simulink model "HybridCarModel"  (R2023a)
settings: Solver=VariableStepAuto  StartTime=0.0  StopTime=10.0  RelTol=1e-3
model workspace (MAT data in the model file):
  Aeff = Simulink.Parameter
  Aeff.Value = 0.0314159265359
  Aeff.DataType = 'double'
  Aeff.Complexity = 'real'
  Aeff.Dimensions = [1 1]
  Af = Simulink.Parameter
  Af.Value = 2.46
  Af.DataType = 'double'
  Af.Complexity = 'real'
  Af.Dimensions = [1 1]
  BattCapInit = Simulink.Parameter
  BattCapInit.Value = 3.18
  BattCapInit.DataType = 'double'
  BattCapInit.Complexity = 'real'
  BattCapInit.Dimensions = [1 1]
  BattChargeMax = Simulink.Parameter
  BattChargeMax.Value = 5.3
  BattChargeMax.DataType = 'double'
  BattChargeMax.Complexity = 'real'
  BattChargeMax.Dimensions = [1 1]
  BattTempBp = Simulink.Parameter
  BattTempBp.Value = [243.1 253.1 263.1 273.1 283.1 298.1 313.1]
  BattTempBp.DataType = 'double'
  BattTempBp.Complexity = 'real'
  BattTempBp.Dimensions = [1 7]
  Bx = Simulink.Parameter
  Bx.Value = 10
  Bx.DataType = 'double'
  Bx.Complexity = 'real'
  Bx.Dimensions = [1 1]
  CapLUTBp = Simulink.Parameter
  CapLUTBp.Value = [0 0.01 0.02 0.03 0.04 0.05 0.06 0.07 0.08 0.09 0.1 0.11 0.12 0.13 0.14 0.15 0.16 0.17 0.18 0.19 0.2 0.21 0.22 0.23 0.24 0.25 0.26 0.27 0.28 0.29 0.3 0.31 0.32 0.33 0.34 0.35 0.36 0.37 0.38 0.39 0.4 0.41 0.42 0.43 0.44 0.45 0.46 0.47 0.48 0.49 0.5 0.51 0.52 0.53 0.54 0.55 0.56 0.57 0.58 0.59 0.6 0.61 0.62 0.63 0.64 0.65 0.66 0.67 0.68 0.69 0.7 0.71 0.72 0.73 0.74 0.75 0.76 0.77 0.78 0.79 0.8 0.81 0.82 0.83 0.84 0.85 0.86 0.87 0.88 0.89 0.9 0.91 0.92 0.93 0.94 0.95 0.96 0.97 0.98 0.99 1]
  CapLUTBp.DataType = 'double'
  CapLUTBp.Complexity = 'real'
  CapLUTBp.Dimensions = [1 101]
  CapSOCBp = Simulink.Parameter
  CapSOCBp.Value = [0 0.2 0.4 0.6 0.8 1]
  CapSOCBp.DataType = 'double'
  CapSOCBp.Complexity = 'real'
  CapSOCBp.Dimensions = [1 6]
  CatLightOffTime = Simulink.Parameter
  CatLightOffTime.Value = 0
  CatLightOffTime.DataType = 'double'
  CatLightOffTime.Complexity = 'real'
  CatLightOffTime.Dimensions = [1 1]
  Cd = Simulink.Parameter
  Cd.Value = 0.25
  Cd.DataType = 'double'
  Cd.Complexity = 'real'
  Cd.Dimensions = [1 1]
  Cl = Simulink.Parameter
  Cl.Value = 0.1
  Cl.DataType = 'double'
  Cl.Complexity = 'real'
  Cl.Dimensions = [1 1]
  Cpm = Simulink.Parameter
  Cpm.Value = 0.1
  Cpm.DataType = 'double'
  Cpm.Complexity = 'real'
  Cpm.Dimensions = [1 1]
  Cps = Simulink.Parameter
  Cps.Value = 2
  Cps.DataType = 'double'
  Cps.Complexity = 'real'
  Cps.Dimensions = [1 1]
  CrankSpeed = Simulink.Parameter
  CrankSpeed.Value = 150
  CrankSpeed.DataType = 'double'
  CrankSpeed.Complexity = 'real'
  CrankSpeed.Dimensions = [1 1]
  Cx = Simulink.Parameter
  Cx.Value = 1.65
  Cx.DataType = 'double'
  Cx.Complexity = 'real'
  Cx.Dimensions = [1 1]
  Dx = Simulink.Parameter
  Dx.Value = 1
  Dx.DataType = 'double'
  Dx.Complexity = 'real'
  Dx.Dimensions = [1 1]
  Em = Simulink.Parameter
  Em.Value = [2.8 3.228 3.284 3.361 3.408 3.427 3.472 3.477 3.493 3.504 3.516 3.528 3.537 3.545 3.555 3.561 3.566 3.576 3.587 3.589 3.594 3.6 3.608 3.61 3.616 3.619 3.626 3.632 3.637 3.64 3.645 3.646 3.652 3.655 3.658 3.661 3.664 3.668 3.673 3.678 3.68 3.681 3.686 3.692 3.699 3.702 3.705 3.71 3.717 3.723 3.728 3.733 3.735 3.742 3.749 3.755 3.761 3.768 3.773 3.78 3.791 3.798 3.798 3.814 3.818 3.825 3.841 3.846 3.855 3.863 3.877 3.885 3.894 3.907 3.919 3.926 3.935 3.944 3.954 3.964 3.974 3.988 3.998 4.014 4.029 4.034 4.047 4.065 4.074 4.086 4.097 4.131 4.126 4.138 4.15 4.18 4.174 4.187 4.207 4.231 4.221]
  Em.DataType = 'double'
  Em.Complexity = 'real'
  Em.Dimensions = [1 101]
  EngRevLim = Simulink.Parameter
  EngRevLim.Value = 7000
  EngRevLim.DataType = 'double'
  EngRevLim.Complexity = 'real'
  EngRevLim.Dimensions = [1 1]
  EngStopStartEnable = Simulink.Parameter
  EngStopStartEnable.Value = 1
  EngStopStartEnable.DataType = 'boolean'
  EngStopStartEnable.Complexity = 'real'
  EngStopStartEnable.Dimensions = [1 1]
  EngStopTime = Simulink.Parameter
  EngStopTime.Value = 5
  EngStopTime.DataType = 'auto'
  EngStopTime.Complexity = 'real'
  EngStopTime.Dimensions = [1 1]
  Ex = Simulink.Parameter
  Ex.Value = 0.01
  Ex.DataType = 'double'
  Ex.Complexity = 'real'
  Ex.Dimensions = [1 1]
  FZMAX = Simulink.Parameter
  FZMAX.Value = 6570
  FZMAX.DataType = 'double'
  FZMAX.Complexity = 'real'
  FZMAX.Dimensions = [1 1]
  FZMIN = Simulink.Parameter
  FZMIN.Value = 0
  FZMIN.DataType = 'double'
  FZMIN.Complexity = 'real'
  FZMIN.Dimensions = [1 1]
  Fc = Simulink.Parameter
  Fc.Value = 500
  Fc.DataType = 'double'
  Fc.Complexity = 'real'
  Fc.Dimensions = [1 1]
  FsbF = Simulink.Parameter
  FsbF.Value = [-700000 -7000 -700 0 700 7000 700000]
  FsbF.DataType = 'double'
  FsbF.Complexity = 'real'
  FsbF.Dimensions = [1 7]
  FsbR = Simulink.Parameter
  FsbR.Value = [-700000 -7000 -700 0 700 7000 700000]
  FsbR.DataType = 'double'
  FsbR.Complexity = 'real'
  FsbR.Dimensions = [1 7]
  FskF = Simulink.Parameter
  FskF.Value = [-8928.57142857 -178.571428571 0 357.142857143 535.714285714 9285.71428571]
  FskF.DataType = 'double'
  FskF.Complexity = 'real'
  FskF.Dimensions = [1 6]
  FskR = Simulink.Parameter
  FskR.Value = [-5357.14285714 -107.142857143 0 214.285714286 321.428571429 5571.42857143]
  FskR.DataType = 'double'
  FskR.Complexity = 'real'
  FskR.Dimensions = [1 6]
  G = Simulink.Parameter
  G.Value = [0 1 2 3 4 5 6]
  G.DataType = 'double'
  G.Complexity = 'real'
  G.Dimensions = [1 7]
  G_o = Simulink.Parameter
  G_o.Value = 1
  G_o.DataType = 'double'
  G_o.Complexity = 'real'
  G_o.Dimensions = [1 1]
  Iyy = Simulink.Parameter
  Iyy.Value = 3000
  Iyy.DataType = 'double'
  Iyy.Complexity = 'real'
  Iyy.Dimensions = [1 1]
  Iyy_Whl = Simulink.Parameter
  Iyy_Whl.Value = 0.8
  Iyy_Whl.DataType = 'double'
  Iyy_Whl.Complexity = 'real'
  Iyy_Whl.Dimensions = [1 1]
  J = Simulink.Parameter
  J.Value = 0.01
  J.DataType = 'double'
  J.Complexity = 'real'
  J.Dimensions = [1 1]
  J1 = Simulink.Parameter
  J1.Value = 0.01
  J1.DataType = 'double'
  J1.Complexity = 'real'
  J1.Dimensions = [1 1]
  J2 = Simulink.Parameter
  J2.Value = 0.01
  J2.DataType = 'double'
  J2.Complexity = 'real'
  J2.Dimensions = [1 1]
  Jd = Simulink.Parameter
  Jd.Value = 0.01
  Jd.DataType = 'double'
  Jd.Complexity = 'real'
  Jd.Dimensions = [1 1]
  Ji = Simulink.Parameter
  Ji.Value = 0.2
  Ji.DataType = 'double'
  Ji.Complexity = 'real'
  Ji.Dimensions = [1 1]
  Jin = Simulink.Parameter
  Jin.Value = 0.05
  Jin.DataType = 'double'
  Jin.Complexity = 'real'
  Jin.Dimensions = [1 1]
  Jin_Cltch = Simulink.Parameter
  Jin_Cltch.Value = 0.2
  Jin_Cltch.DataType = 'double'
  Jin_Cltch.Complexity = 'real'
  Jin_Cltch.Dimensions = [1 1]
  Jin_Cltch2 = Simulink.Parameter
  Jin_Cltch2.Value = 0.01
  Jin_Cltch2.DataType = 'double'
  Jin_Cltch2.Complexity = 'real'
  Jin_Cltch2.Dimensions = [1 1]
  Jout = Simulink.Parameter
  Jout.Value = [0.009 0.01 0.01 0.01 0.01 0.01 0.01]
  Jout.DataType = 'double'
  Jout.Complexity = 'real'
  Jout.Dimensions = [1 7]
  Jout_Cltch = Simulink.Parameter
  Jout_Cltch.Value = 0.01
  Jout_Cltch.DataType = 'double'
  Jout_Cltch.Complexity = 'real'
  Jout_Cltch.Dimensions = [1 1]
  Jout_Cltch2 = Simulink.Parameter
  Jout_Cltch2.Value = 0.05
  Jout_Cltch2.DataType = 'double'
  Jout_Cltch2.Complexity = 'real'
  Jout_Cltch2.Dimensions = [1 1]
  Jt = Simulink.Parameter
  Jt.Value = 0.01
  Jt.DataType = 'double'
  Jt.Complexity = 'real'
  Jt.Dimensions = [1 1]
  Jw1 = Simulink.Parameter
  Jw1.Value = 0.01
  Jw1.DataType = 'double'
  Jw1.Complexity = 'real'
  Jw1.Dimensions = [1 1]
  Jw2 = Simulink.Parameter
  Jw2.Value = 0.01
  Jw2.DataType = 'double'
  Jw2.Complexity = 'real'
  Jw2.Dimensions = [1 1]
  K_c = Simulink.Parameter
  K_c.Value = 10000
  K_c.DataType = 'double'
  K_c.Complexity = 'real'
  K_c.Dimensions = [1 1]
  Lrel = Simulink.Parameter
  Lrel.Value = 0.15
  Lrel.DataType = 'double'
  Lrel.Complexity = 'real'
  Lrel.Dimensions = [1 1]
  Mass = Simulink.Parameter
  Mass.Value = 1623
  Mass.DataType = 'double'
  Mass.Complexity = 'real'
  Mass.Dimensions = [1 1]
  N = Simulink.Parameter
  N.Value = [1 4.212 2.637 1.8 1.386 1 0.772]
  N.DataType = 'double'
  N.Complexity = 'real'
  N.Dimensions = [1 7]
  NCyl = Simulink.Parameter
  NCyl.Value = 4
  NCyl.DataType = 'double'
  NCyl.Complexity = 'real'
  NCyl.Dimensions = [1 1]
  NF = Simulink.Parameter
  NF.Value = 2
  NF.DataType = 'double'
  NF.Complexity = 'real'
  NF.Dimensions = [1 1]
  NR = Simulink.Parameter
  NR.Value = 2
  NR.DataType = 'double'
  NR.Complexity = 'real'
  NR.Dimensions = [1 1]
  N_P4 = Simulink.Parameter
  N_P4.Value = 4.1
  N_P4.DataType = 'double'
  N_P4.Complexity = 'real'
  N_P4.Dimensions = [1 1]
  N_idle = Simulink.Parameter
  N_idle.Value = 750
  N_idle.DataType = 'double'
  N_idle.Complexity = 'real'
  N_idle.Dimensions = [1 1]
  Ndiff = Simulink.Parameter
  Ndiff.Value = 3.32
  Ndiff.DataType = 'double'
  Ndiff.Complexity = 'real'
  Ndiff.Dimensions = [1 1]
  Ndiff_P4 = Simulink.Parameter
  Ndiff_P4.Value = 4.1
  Ndiff_P4.DataType = 'double'
  Ndiff_P4.Complexity = 'real'
  Ndiff_P4.Dimensions = [1 1]
  Ndisk = Simulink.Parameter
  Ndisk.Value = 1
  Ndisk.DataType = 'double'
  Ndisk.Complexity = 'real'
  Ndisk.Dimensions = [1 1]
  Ndisks = Simulink.Parameter
  Ndisks.Value = 4
  Ndisks.DataType = 'double'
  Ndisks.Complexity = 'real'
  Ndisks.Dimensions = [1 1]
  Np = Simulink.Parameter
  Np.Value = 1
  Np.DataType = 'double'
  Np.Complexity = 'real'
  Np.Dimensions = [1 1]
  Ns = Simulink.Parameter
  Ns.Value = 72
  Ns.DataType = 'double'
  Ns.Complexity = 'real'
  Ns.Dimensions = [1 1]
  Pabs = Simulink.Parameter
  Pabs.Value = 101325
  Pabs.DataType = 'double'
  Pabs.Complexity = 'real'
  Pabs.Dimensions = [1 1]
  Plimit = Simulink.Parameter
  Plimit.Value = 30000
  Plimit.DataType = 'double'
  Plimit.Complexity = 'real'
  Plimit.Dimensions = [1 1]
  Press = Simulink.Parameter
  Press.Value = 7000000
  Press.DataType = 'double'
  Press.Complexity = 'real'
  Press.Dimensions = [1 1]
  Pstd = Simulink.Parameter
  Pstd.Value = 101325
  Pstd.DataType = 'double'
  Pstd.Complexity = 'real'
  Pstd.Dimensions = [1 1]
  RInt = Simulink.Parameter
  RInt.Value = [0.008846  0.009319  0.009027  0.00847  0.01032  0.01314; 0.006389  0.006554  0.005553  0.005525  0.006043  0.007805; 0.004364  0.004101  0.00406  0.003452  0.003846  0.004517; 0.002031  0.002563  0.002532  0.00246  0.002716  0.003047; 0.001443  0.001825  0.001795  0.001778  0.001924  0.002234; 0.0005603  0.0007192  0.0006887  0.0007557  0.0007355  0.001014; 0.001028  0.001338  0.001  0.001536  0.001546  0.002789]
  RInt.DataType = 'double'
  RInt.Complexity = 'real'
  RInt.Dimensions = [7 6]
  Rair = Simulink.Parameter
  Rair.Value = 287
  Rair.DataType = 'double'
  Rair.Complexity = 'real'
  Rair.Dimensions = [1 1]
  Re = Simulink.Parameter
  Re.Value = 0.327
  Re.DataType = 'double'
  Re.Complexity = 'real'
  Re.Dimensions = [1 1]
  Reff = Simulink.Parameter
  Reff.Value = 0.11
  Reff.DataType = 'double'
  Reff.Complexity = 'real'
  Reff.Dimensions = [1 1]
  Reff_LSD = Simulink.Parameter
  Reff_LSD.Value = 0.2
  Reff_LSD.DataType = 'double'
  Reff_LSD.Complexity = 'real'
  Reff_LSD.Dimensions = [1 1]
  Rm = Simulink.Parameter
  Rm.Value = 0.15
  Rm.DataType = 'double'
  Rm.Complexity = 'real'
  Rm.Dimensions = [1 1]
  Sinj = Simulink.Parameter
  Sinj.Value = 6.45161290323
  Sinj.DataType = 'double'
  Sinj.Complexity = 'real'
  Sinj.Dimensions = [1 1]
  T = Simulink.Parameter
  T.Value = 300
  T.DataType = 'double'
  T.Complexity = 'real'
  T.Dimensions = [1 1]
  T_eff_bp = Simulink.Parameter
  T_eff_bp.Value = [0 20 40 60 80 100 120 140 160 180 200]
  T_eff_bp.DataType = 'double'
  T_eff_bp.Complexity = 'real'
  T_eff_bp.Dimensions = [1 11]
  T_t = Simulink.Parameter
  T_t.Value = [200 200 200 200 190.9859317 143.2394488 114.591559 95.49296586 81.85111359 71.61972439 63.66197724 57.29577951 52.08707228 47.74648293]
  T_t.DataType = 'double'
  T_t.Complexity = 'real'
  T_t.Dimensions = [1 14]
  Tc = Simulink.Parameter
  Tc.Value = 0.02
  Tc.DataType = 'double'
  Tc.Complexity = 'real'
  Tc.Dimensions = [1 1]
  Temp_bpts = Simulink.Parameter
  Temp_bpts.Value = [313 358]
  Temp_bpts.DataType = 'double'
  Temp_bpts.Complexity = 'real'
  Temp_bpts.Dimensions = [1 2]
  Trq_bpts = Simulink.Parameter
  Trq_bpts.Value = [25 50 75 100 150 200 250]
  Trq_bpts.DataType = 'double'
  Trq_bpts.Complexity = 'real'
  Trq_bpts.Dimensions = [1 7]
  Ts = Simulink.Parameter
  Ts.Value = 0.01
  Ts.DataType = 'auto'
  Ts.Complexity = 'real'
  Ts.Dimensions = [1 1]
  Tstd = Simulink.Parameter
  Tstd.Value = 293.15
  Tstd.DataType = 'double'
  Tstd.Complexity = 'real'
  Tstd.Dimensions = [1 1]
  UNLOADED_RADIUS = Simulink.Parameter
  UNLOADED_RADIUS.Value = 0.336
  UNLOADED_RADIUS.DataType = 'double'
  UNLOADED_RADIUS.Complexity = 'real'
  UNLOADED_RADIUS.Dimensions = [1 1]
  VXLOW = Simulink.Parameter
  VXLOW.Value = 2
  VXLOW.DataType = 'double'
  VXLOW.Complexity = 'real'
  VXLOW.Dimensions = [1 1]
  Vd = Simulink.Parameter
  Vd.Value = 0.0015
  Vd.DataType = 'double'
  Vd.Complexity = 'real'
  Vd.Dimensions = [1 1]
  Vinit = Simulink.Parameter
  Vinit.Value = 650
  Vinit.DataType = 'double'
  Vinit.Complexity = 'real'
  Vinit.Dimensions = [1 1]
  aMy = Simulink.Parameter
  aMy.Value = 0.01
  aMy.DataType = 'double'
  aMy.Complexity = 'real'
  aMy.Dimensions = [1 1]
  a_CG = Simulink.Parameter
  a_CG.Value = 1.09
  a_CG.DataType = 'double'
  a_CG.Complexity = 'real'
  a_CG.Dimensions = [1 1]
  afr_stoich = Simulink.Parameter
  afr_stoich.Value = 14.6
  afr_stoich.DataType = 'double'
  afr_stoich.Complexity = 'real'
  afr_stoich.Dimensions = [1 1]
  alphaMy = Simulink.Parameter
  alphaMy.Value = 0
  alphaMy.DataType = 'double'
  alphaMy.Complexity = 'real'
  alphaMy.Dimensions = [1 1]
  b = Simulink.Parameter
  b.Value = 400
  b.DataType = 'auto'
  b.Complexity = 'real'
  b.Dimensions = [1 1]
  b1 = Simulink.Parameter
  b1.Value = 100
  b1.DataType = 'double'
  b1.Complexity = 'real'
  b1.Dimensions = [1 1]
  b1_g = Simulink.Parameter
  b1_g.Value = 0.001
  b1_g.DataType = 'double'
  b1_g.Complexity = 'real'
  b1_g.Dimensions = [1 1]
  b2 = Simulink.Parameter
  b2.Value = 100
  b2.DataType = 'double'
  b2.Complexity = 'real'
  b2.Dimensions = [1 1]
  b2_g = Simulink.Parameter
  b2_g.Value = 0.001
  b2_g.DataType = 'double'
  b2_g.Complexity = 'real'
  b2_g.Dimensions = [1 1]
  bMy = Simulink.Parameter
  bMy.Value = 0
  bMy.DataType = 'double'
  bMy.Complexity = 'real'
  bMy.Dimensions = [1 1]
  b_CG = Simulink.Parameter
  b_CG.Value = 1.7
  b_CG.DataType = 'double'
  b_CG.Complexity = 'real'
  b_CG.Dimensions = [1 1]
  b_J = Simulink.Parameter
  b_J.Value = 0.001
  b_J.DataType = 'double'
  b_J.Complexity = 'real'
  b_J.Dimensions = [1 1]
  bd = Simulink.Parameter
  bd.Value = 0.001
  bd.DataType = 'double'
  bd.Complexity = 'real'
  bd.Dimensions = [1 1]
  betaMy = Simulink.Parameter
  betaMy.Value = 1
  betaMy.DataType = 'double'
  betaMy.Complexity = 'real'
  betaMy.Dimensions = [1 1]
  bi = Simulink.Parameter
  bi.Value = 0.001
  bi.DataType = 'double'
  bi.Complexity = 'real'
  bi.Dimensions = [1 1]
  bin = Simulink.Parameter
  bin.Value = 0.003
  bin.DataType = 'double'
  bin.Complexity = 'real'
  bin.Dimensions = [1 1]
  bin_Cltch = Simulink.Parameter
  bin_Cltch.Value = 0.003
  bin_Cltch.DataType = 'double'
  bin_Cltch.Complexity = 'real'
  bin_Cltch.Dimensions = [1 1]
  bout = Simulink.Parameter
  bout.Value = [0.003 0.003 0.003 0.003 0.003 0.003 0.003]
  bout.DataType = 'double'
  bout.Complexity = 'real'
  bout.Dimensions = [1 7]
  bout_Cltch = Simulink.Parameter
  bout_Cltch.Value = 0.003
  bout_Cltch.DataType = 'double'
  bout_Cltch.Complexity = 'real'
  bout_Cltch.Dimensions = [1 1]
  br = Simulink.Parameter
  br.Value = 0.001
  br.DataType = 'double'
  br.Complexity = 'real'
  br.Dimensions = [1 1]
  bt = Simulink.Parameter
  bt.Value = 0.001
  bt.DataType = 'double'
  bt.Complexity = 'real'
  bt.Dimensions = [1 1]
  bw1 = Simulink.Parameter
  bw1.Value = 0.001
  bw1.DataType = 'double'
  bw1.Complexity = 'real'
  bw1.Dimensions = [1 1]
  bw2 = Simulink.Parameter
  bw2.Value = 0.001
  bw2.DataType = 'double'
  bw2.Complexity = 'real'
  bw2.Dimensions = [1 1]
  cMy = Simulink.Parameter
  cMy.Value = 0
  cMy.DataType = 'double'
  cMy.Complexity = 'real'
  cMy.Dimensions = [1 1]
  calEngVar.core.f_lcmd = [0 0.191691264236 0.286571334918 0.358602176328 0.434951284075 0.517809236578 0.591334464387 0.61481465749 0.61481465749 0.61481465749 0.61481465749 0.61481465749 ... (315 elements, 21x15)]
  calEngVar.core.f_tap = [0 0.526932471367 0.769562920372 0.98216383526 1.23343075188 1.55068263762 2.00046959085 2.58135491039 2.62499999998 2.62499999998 2.62499999998 2.62499999998 ... (315 elements, 21x15)]
  calEngVar.core.f_wap = [100 100 100 100 100 100 100 100 100 100 100 100 ... (315 elements, 21x15)]
  calEngVar.coreNA.f_lcmd = [0 0.191673794236 0.286480813868 0.358962317026 0.435201371684 0.516947124026 0.591296592004 0.593111529261 0.593111636908 0.593111710683 0.593111746853 0.593111755564 ... (315 elements, 21x15)]
  calEngVar.coreNA.f_tap = [0 0.527345242717 0.765291484509 0.982320090188 1.22180302541 1.45741485748 1.74956862606 2 2 2 2 2 ... (315 elements, 21x15)]
  calEngVar.coreNA.f_wap = [100 100 100 100 100 100 100 100 100 100 100 100 ... (315 elements, 21x15)]
  calEngVar.coreV.f_lcmd = [0 0.191421421753 0.286577353388 0.358588536544 0.434930146898 0.517765102071 0.591331638707 0.613375617301 0.613375617301 0.613375617301 0.613375617301 0.613375617301 ... (315 elements, 21x15)]
  calEngVar.coreV.f_tap = [0 0.527863235448 0.770830749421 0.984101116219 1.23615501042 1.5569451281 2.00979487112 2.59646979725 2.62499999998 2.62499999998 2.62499999998 2.62499999998 ... (315 elements, 21x15)]
  calEngVar.coreV.f_wap = [100 100 100 100 100 100 100 100 100 100 100 100 ... (315 elements, 21x15)]
  calEngVar.coreV2.f_lcmd = [0 0.194061751813 0.287076886738 0.359012181592 0.434856378234 0.517000734831 0.591338874186 0.631368544619 0.631368695337 0.631369347621 0.631369911122 0.631370243827 ... (315 elements, 21x15)]
  calEngVar.coreV2.f_tap = [0 0.393432535935 0.590588347082 0.770979860518 0.943173243753 1.202063296 1.55415454297 2.04859040123 2.24999782819 2.24999782819 2.24999782819 2.24999782819 ... (315 elements, 21x15)]
  calEngVar.coreV2.f_wap = [100 100 100 100 100 100 100 100 100 100 100 100 ... (315 elements, 21x15)]
  calEngVar.coreVNA.f_lcmd = [0 0.191673794234 0.286480814132 0.358962317057 0.435201376817 0.516947124415 0.5912965923 0.593111627658 0.593111729822 0.593111798315 0.593111829983 0.593111834102 ... (315 elements, 21x15)]
  calEngVar.coreVNA.f_tap = [0 0.527345232148 0.765291599327 0.982320090386 1.22180321714 1.45741495752 1.74956861419 2 2 2 2 2 ... (315 elements, 21x15)]
  calEngVar.coreVNA.f_wap = [100 100 100 100 100 100 100 100 100 100 100 100 ... (315 elements, 21x15)]
  disk_abore = Simulink.Parameter
  disk_abore.Value = 0.05
  disk_abore.DataType = 'double'
  disk_abore.Complexity = 'real'
  disk_abore.Dimensions = [1 1]
  domega_o = Simulink.Parameter
  domega_o.Value = 0
  domega_o.DataType = 'double'
  domega_o.Complexity = 'real'
  domega_o.Dimensions = [1 1]
  dw = Simulink.Parameter
  dw.Value = [0 10 20 40 60 80 100]
  dw.DataType = 'double'
  dw.Complexity = 'real'
  dw.Dimensions = [1 7]
  dzdotsF = Simulink.Parameter
  dzdotsF.Value = [-10 -1 -0.1 0 0.1 1 10]
  dzdotsF.DataType = 'double'
  dzdotsF.Complexity = 'real'
  dzdotsF.Dimensions = [1 7]
  dzdotsR = Simulink.Parameter
  dzdotsR.Value = [-10 -1 -0.1 0 0.1 1 10]
  dzdotsR.DataType = 'double'
  dzdotsR.Complexity = 'real'
  dzdotsR.Dimensions = [1 7]
  dzsF = Simulink.Parameter
  dzsF.Value = [-0.005 -0.0001 0 0.2 0.2001 0.2051]
  dzsF.DataType = 'double'
  dzsF.Complexity = 'real'
  dzsF.Dimensions = [1 6]
  dzsR = Simulink.Parameter
  dzsR.Value = [-0.005 -0.0001 0 0.2 0.2001 0.2051]
  dzsR.DataType = 'double'
  dzsR.Complexity = 'real'
  dzsR.Dimensions = [1 6]
  eff = Simulink.Parameter
  eff.Value = 98
  eff.DataType = 'double'
  eff.Complexity = 'real'
  eff.Dimensions = [1 1]
  efficiency_table = Simulink.Parameter
  efficiency_table.Value = [52  78  80  82  82  80  78  78  76  74  70; 52  78  80  82  82  80  78  78  76  74  70; 52  78  84  86  86  86  86  84  84  82  82; 52  80  86  86  88  88  88  86  86  84  84; 52  80  86  88  88  88  88  88  86  86  86; 52  80  86  88  90  90  90  90  88  88  88; 52  82  88  90  91  91  92  92  92  91  91; 52  82  88  91  91  92  93  93  93  93  93; 52  84  90  92  92  93  93  93  93  93  93; 62  86  91  93  93  93  93  93  93  93  93; 66  86  91  93  93  93  93  93  93  93  93; 70  86  92  93  93  93  93  93  93  93  93; 70  86  92  93  93  93  93  93  93  93  93; 72  86  91  93  93  93  93  93  93  93  93]
  efficiency_table.DataType = 'double'
  efficiency_table.Complexity = 'real'
  efficiency_table.Dimensions = [14 11]
  eta = Simulink.Parameter
  eta.Value = [0.95 0.95 0.95 0.95 0.95 0.95 0.95]
  eta.DataType = 'double'
  eta.Complexity = 'real'
  eta.Dimensions = [1 7]
  eta_diff = Simulink.Parameter
  eta_diff.Value = 0.98
  eta_diff.DataType = 'double'
  eta_diff.Complexity = 'real'
  eta_diff.Dimensions = [1 1]
  eta_tbl = Simulink.Parameter
  eta_tbl.Value = [0.766 0.766 0.766 0.766 0.766 0.766 0.766 0.766 0.766 0.766 0.766 0.766 ... (1078 elements, 7x11x7x2)]
  eta_tbl.DataType = 'double'
  eta_tbl.Complexity = 'real'
  eta_tbl.Dimensions = [7 11 7 2]
  f_cp_ld_bpt = Simulink.Parameter
  f_cp_ld_bpt.Value = [0 0.2 0.275 0.35 0.425 0.5 0.575 0.65 0.725 0.8 0.875 0.95 1.025 1.1 1.175 1.25]
  f_cp_ld_bpt.DataType = 'double'
  f_cp_ld_bpt.Complexity = 'real'
  f_cp_ld_bpt.Dimensions = [1 16]
  f_cp_n_bpt = Simulink.Parameter
  f_cp_n_bpt.Value = [750 1053.57142857 1357.14285714 1660.71428571 1964.28571429 2267.85714286 2571.42857143 2875 3178.57142857 3482.14285714 3785.71428571 4089.28571429 4392.85714286 4696.42857143 5000]
  f_cp_n_bpt.DataType = 'double'
  f_cp_n_bpt.Complexity = 'real'
  f_cp_n_bpt.Dimensions = [1 15]
  f_del_sa_bpt = Simulink.Parameter
  f_del_sa_bpt.Value = [0 0.75 1.5 2.25 3 3.75 4.5 5.25 6 6.75 7.5 8.25 9 9.75 10.5 11.25 12 12.75 13.5 14.25 15 15.75 16.5 17.25 18 18.75 19.5 20.25 21 21.75 22.5 23.25 24 24.75 25.5 26.25 27 27.75 28.5 29.25 30 30.75 31.5 32.25 33 33.75 34.5 35.25 36 36.75 37.5 38.25 39 39.75 40.5 41.25 42 42.75 43.5 44.25 45 45.75 46.5 47.25 48]
  f_del_sa_bpt.DataType = 'double'
  f_del_sa_bpt.Complexity = 'real'
  f_del_sa_bpt.Dimensions = [1 65]
  f_ecp = Simulink.Parameter
  f_ecp.Value = [0 0 7.19012817097 15.3709456879 19.1470470057 19.0854874367 13.5819971805 0 0 0 0 0 ... (240 elements, 16x15)]
  f_ecp.DataType = 'double'
  f_ecp.Complexity = 'real'
  f_ecp.Dimensions = [16 15]
  f_egr_areapct_cmd = Simulink.Parameter
  f_egr_areapct_cmd.Value = [0 3.448 6.897 10.34 13.79 17.24 20.69 24.14 27.59 31.03 34.48 37.93 ... (600 elements, 30x20)]
  f_egr_areapct_cmd.DataType = 'double'
  f_egr_areapct_cmd.Complexity = 'real'
  f_egr_areapct_cmd.Dimensions = [30 20]
  f_egr_areapct_nrmlzdflow_bpt = Simulink.Parameter
  f_egr_areapct_nrmlzdflow_bpt.Value = [0 0.03448 0.06897 0.1034 0.1379 0.1724 0.2069 0.2414 0.2759 0.3103 0.3448 0.3793 0.4138 0.4483 0.4828 0.5172 0.5517 0.5862 0.6207 0.6552 0.6897 0.7241 0.7586 0.7931 0.8276 0.8621 0.8966 0.931 0.9655 1]
  f_egr_areapct_nrmlzdflow_bpt.DataType = 'double'
  f_egr_areapct_nrmlzdflow_bpt.Complexity = 'real'
  f_egr_areapct_nrmlzdflow_bpt.Dimensions = [1 30]
  f_egr_areapct_pr_bpt = Simulink.Parameter
  f_egr_areapct_pr_bpt.Value = [0.5; 0.5263; 0.5526; 0.5789; 0.6053; 0.6316; 0.6579; 0.6842; 0.7105; 0.7368; 0.7632; 0.7895; 0.8158; 0.8421; 0.8684; 0.8947; 0.9211; 0.9474; 0.9737; 1]
  f_egr_areapct_pr_bpt.DataType = 'double'
  f_egr_areapct_pr_bpt.Complexity = 'real'
  f_egr_areapct_pr_bpt.Dimensions = [20 1]
  f_egr_max_stdflow = Simulink.Parameter
  f_egr_max_stdflow.Value = [74.87 74.87 74.74 74.39 73.81 72.98 71.91 70.58 68.97 67.06 64.84 62.25 59.27 55.81 51.79 47.07 36.33 24.22 12.11 0]
  f_egr_max_stdflow.DataType = 'double'
  f_egr_max_stdflow.Complexity = 'real'
  f_egr_max_stdflow.Dimensions = [1 20]
  f_egr_stdflow = Simulink.Parameter
  f_egr_stdflow.Value = [0 3.743 7.487 11.23 14.97 18.72 22.46 26.2 29.95 33.69 37.43 41.18 ... (420 elements, 21x20)]
  f_egr_stdflow.DataType = 'double'
  f_egr_stdflow.Complexity = 'real'
  f_egr_stdflow.Dimensions = [21 20]
  f_egr_stdflow_egrap_bpt = Simulink.Parameter
  f_egr_stdflow_egrap_bpt.Value = [0; 5; 10; 15; 20; 25; 30; 35; 40; 45; 50; 55; 60; 65; 70; 75; 80; 85; 90; 95; 100]
  f_egr_stdflow_egrap_bpt.DataType = 'double'
  f_egr_stdflow_egrap_bpt.Complexity = 'real'
  f_egr_stdflow_egrap_bpt.Dimensions = [21 1]
  f_egr_stdflow_pr_bpt = Simulink.Parameter
  f_egr_stdflow_pr_bpt.Value = [0.5; 0.5263; 0.5526; 0.5789; 0.6053; 0.6316; 0.6579; 0.6842; 0.7105; 0.7368; 0.7632; 0.7895; 0.8158; 0.8421; 0.8684; 0.8947; 0.9211; 0.9474; 0.9737; 1]
  f_egr_stdflow_pr_bpt.DataType = 'double'
  f_egr_stdflow_pr_bpt.Complexity = 'real'
  f_egr_stdflow_pr_bpt.Dimensions = [20 1]
  f_egrpct_cmd = Simulink.Parameter
  f_egrpct_cmd.Value = [0  0  0  0  0  0  0  0  0  0  0  0  0  0  0; 0  0  0  0  0  0  0  0  0  0  0  0  0  0  0; 0  0  0  0  0  0  0  0  0  0  0  0  0  0  0; 0  0  0  0  0  0  0  0  0  0  0  0  0  0  0; 0  0  0  0  0  0  0  0  0  0  0  0  0  0  0; 0  0  0  0  0  0  0  0  0  0  0  0  0  0  0; 0  0  0  0  0  0  0  0  0  0  0  0  0  0  0; 0  0  0  0  0  0  0  0  0  0  0  0  0  0  0; 0  0  0  0  0  0  0  0  0  0  0  0  0  0  0; 0  0  0  0  0  0  0  0  0  0  0  0  0  0  0; 0  0  0  0  0  0  0  0  0  0  0  0  0  0  0; 0  0  0  0  0  0  0  0  0  0  0  0  0  0  0; 0  0  0  0  0  0  0  0  0  0  0  0  0  0  0; 0  0  0  0  0  0  0  0  0  0  0  0  0  0  0; 0  0  0  0  0  0  0  0  0  0  0  0  0  0  0; 0  0  0  0  0  0  0  0  0  0  0  0  0  0  0]
  f_egrpct_cmd.DataType = 'double'
  f_egrpct_cmd.Complexity = 'real'
  f_egrpct_cmd.Dimensions = [16 15]
  f_egrpct_ld_bpt = Simulink.Parameter
  f_egrpct_ld_bpt.Value = [0 0.2 0.275 0.35 0.425 0.5 0.575 0.65 0.725 0.8 0.875 0.95 1.025 1.1 1.175 1.25]
  f_egrpct_ld_bpt.DataType = 'double'
  f_egrpct_ld_bpt.Complexity = 'real'
  f_egrpct_ld_bpt.Dimensions = [1 16]
  f_egrpct_n_bpt = Simulink.Parameter
  f_egrpct_n_bpt.Value = [750 1054 1357 1661 1964 2268 2571 2875 3179 3482 3786 4089 4393 4696 5000]
  f_egrpct_n_bpt.DataType = 'double'
  f_egrpct_n_bpt.Complexity = 'real'
  f_egrpct_n_bpt.Dimensions = [1 15]
  f_fric_temp_bpt = Simulink.Parameter
  f_fric_temp_bpt.Value = [274 276 278 280 282 284 286 288 290 292 294 296 298 300 302 304 306 308 310 312 314 316 318 320 322 324 326 328 330 332 334 336 338 340 342 344 346 348 350 352 354 356 358 360 362 364 366 368 370 372 374 376 378 380]
  f_fric_temp_bpt.DataType = 'double'
  f_fric_temp_bpt.Complexity = 'real'
  f_fric_temp_bpt.Dimensions = [1 54]
  f_fric_temp_mod = Simulink.Parameter
  f_fric_temp_mod.Value = [3.96 3.22 2.56 2.26 2.11 2 1.9 1.83 1.76 1.7 1.65 1.6 1.55 1.49 1.44 1.41 1.38 1.35 1.32 1.3 1.27 1.25 1.24 1.21 1.2 1.18 1.16 1.15 1.13 1.12 1.11 1.1 1.09 1.08 1.07 1.06 1.05 1.05 1.04 1.03 1.02 1.02 1.01 1.01 1 1 1 0.999 0.997 0.995 0.993 0.991 0.989 0.987]
  f_fric_temp_mod.DataType = 'double'
  f_fric_temp_mod.Complexity = 'real'
  f_fric_temp_mod.Dimensions = [1 54]
  f_icp = Simulink.Parameter
  f_icp.Value = [0 0 1 1.09273642197 2.29409401139 3.54274371837 0.947749647567 0 0 0 0 0 ... (240 elements, 16x15)]
  f_icp.DataType = 'double'
  f_icp.Complexity = 'real'
  f_icp.Dimensions = [16 15]
  f_intksys_stdflow_bpt = Simulink.Parameter
  f_intksys_stdflow_bpt.Value = [0 29.67 59.34 89.01 117.8 144.1 155.7 166 175.2 183.3 190.7 197 202.7 207.7 212.2 216.1 219.4 222.2 224.5 226.4]
  f_intksys_stdflow_bpt.DataType = 'double'
  f_intksys_stdflow_bpt.Complexity = 'real'
  f_intksys_stdflow_bpt.Dimensions = [1 20]
  f_intksys_stdflow_pr = Simulink.Parameter
  f_intksys_stdflow_pr.Value = [1 0.9789 0.9579 0.9368 0.9158 0.8947 0.8737 0.8526 0.8316 0.8105 0.7895 0.7684 0.7474 0.7263 0.7053 0.6842 0.6632 0.6421 0.6211 0.6]
  f_intksys_stdflow_pr.DataType = 'double'
  f_intksys_stdflow_pr.Complexity = 'real'
  f_intksys_stdflow_pr.Dimensions = [1 20]
  f_lamcmd = Simulink.Parameter
  f_lamcmd.Value = [1  1  1  1  1  1  1  1  1  1  1  1  1  1  1; 1  1  1  1  1  1  1  1  1  1  1  1  1  1  1; 1  1  1  1  1  1  1  1  1  1  1  1  1  1  1; 1  1  1  1  1  1  1  1  1  1  1  1  1  1  1; 1  1  1  1  1  1  1  1  1  1  1  1  1  1  1; 1  1  1  1  1  1  1  1  1  1  1  1  1  1  1; 1  1  1  1  1  1  1  1  1  1  1  1  1  1  1; 1  1  1  1  1  1  1  1  1  1  1  1  1  1  1; 1  1  1  1  1  1  1  1  1  1  1  1  1  1  1; 1  1  1  1  1  1  1  1  1  1  1  1  1  1  1; 1  1  1  1  1  1  1  1  1  1  1  1  1  1  0.978833376279; 1  1  1  1  1  0.994115442909  1  0.972947102204  0.980523305065  0.999379925377  1  0.999606769395  0.999730304812  0.995941175028  0.966904774685; 1  1  1  0.94651624294  1  0.952506105741  0.994491417815  0.906466250495  0.924122061249  0.974767007025  0.985748891861  0.982416523617  0.992900047913  0.942109771144  0.941787575943; 1  1  1  0.942  0.937279637266  0.910896768573  0.929830385386  0.839985398785  0.854904769548  0.889462296842  0.92380217143  0.919912974116  0.958707785886  0.945711085936  0.914402970615; 1  1  1  0.942  0.902  0.869287431405  0.865169352957  0.81  0.824  0.812  0.837314196571  0.85940898562  0.888506841156  0.882667105929  0.87548189152; 1  1  1  0.942  0.902  0.846  0.824  0.81  0.824  0.812  0.826  0.818  0.815209011399  0.813810193086  0.836]
  f_lamcmd.DataType = 'double'
  f_lamcmd.Complexity = 'real'
  f_lamcmd.Dimensions = [16 15]
  f_lamcmd_ld_bpt = Simulink.Parameter
  f_lamcmd_ld_bpt.Value = [0 0.2 0.275 0.35 0.425 0.5 0.575 0.65 0.725 0.8 0.875 0.95 1.025 1.1 1.175 1.25]
  f_lamcmd_ld_bpt.DataType = 'double'
  f_lamcmd_ld_bpt.Complexity = 'real'
  f_lamcmd_ld_bpt.Dimensions = [1 16]
  f_lamcmd_n_bpt = Simulink.Parameter
  f_lamcmd_n_bpt.Value = [750 1053.57142857 1357.14285714 1660.71428571 1964.28571429 2267.85714286 2571.42857143 2875 3178.57142857 3482.14285714 3785.71428571 4089.28571429 4392.85714286 4696.42857143 5000]
  f_lamcmd_n_bpt.DataType = 'double'
  f_lamcmd_n_bpt.Complexity = 'real'
  f_lamcmd_n_bpt.Dimensions = [1 15]
  f_lcmd = Simulink.Parameter
  f_lcmd.Value = [0 0.191691264236 0.286571334918 0.358602176328 0.434951284075 0.517809236578 0.591334464387 0.61481465749 0.61481465749 0.61481465749 0.61481465749 0.61481465749 ... (315 elements, 21x15)]
  f_lcmd.DataType = 'double'
  f_lcmd.Complexity = 'real'
  f_lcmd.Dimensions = [21 15]
  f_lcmd_n_bpt = Simulink.Parameter
  f_lcmd_n_bpt.Value = [750 1053.57142857 1357.14285714 1660.71428571 1964.28571429 2267.85714286 2571.42857143 2875 3178.57142857 3482.14285714 3785.71428571 4089.28571429 4392.85714286 4696.42857143 5000]
  f_lcmd_n_bpt.DataType = 'double'
  f_lcmd_n_bpt.Complexity = 'real'
  f_lcmd_n_bpt.Dimensions = [1 15]
  f_lcmd_tq_bpt = Simulink.Parameter
  f_lcmd_tq_bpt.Value = [0 15 26.3157894737 37.6315789474 48.9473684211 60.2631578947 71.5789473684 82.8947368421 94.2105263158 105.526315789 116.842105263 128.157894737 139.473684211 150.789473684 162.105263158 173.421052632 184.736842105 196.052631579 207.368421053 218.684210526 230]
  f_lcmd_tq_bpt.DataType = 'double'
  f_lcmd_tq_bpt.Complexity = 'real'
  f_lcmd_tq_bpt.Dimensions = [1 21]
  f_m_lam = Simulink.Parameter
  f_m_lam.Value = [0.94128 0.95565 0.97001 0.98437 0.99008 1.0004 0.97527 0.9549 0.92612 0.89735 0]
  f_m_lam.DataType = 'double'
  f_m_lam.Complexity = 'real'
  f_m_lam.Dimensions = [1 11]
  f_m_lam_bpt = Simulink.Parameter
  f_m_lam_bpt.Value = [0.65 0.7 0.75 0.8 0.85 0.9 0.95 1 1.05 1.1 2]
  f_m_lam_bpt.DataType = 'double'
  f_m_lam_bpt.Complexity = 'real'
  f_m_lam_bpt.Dimensions = [1 11]
  f_m_sa = Simulink.Parameter
  f_m_sa.Value = [1.0019 0.9988 0.9953 0.99173 0.98811 0.98441 0.98065 0.97682 0.97293 0.96897 0.96493 0.96083 0.95666 0.95242 0.94811 0.94373 0.93927 0.93475 0.93015 0.92548 0.92074 0.91592 0.91104 0.90608 0.90105 0.89594 0.89076 0.88551 0.88019 0.8748 0.86933 0.86379 0.85818 0.8525 0.84675 0.84093 0.83503 0.82907 0.82303 0.81693 0.81075 0.80451 0.79819 0.79181 0.78536 0.77884 0.77226 0.7656 0.75888 0.75209 0.74524 0.73832 0.73134 0.72429 0.71717 0.70999 0.70275 0.69682 0.68949 0.68303 0.67548 0.67037 0.66525 0.66014 0.65503]
  f_m_sa.DataType = 'double'
  f_m_sa.Complexity = 'real'
  f_m_sa.Dimensions = [1 65]
  f_mdot_air_corr = Simulink.Parameter
  f_mdot_air_corr.Value = [1.02156051768 1.00597426471 0.989411677851 1.0033499089 0.984591437857 0.988509040623 1.0326198627 1.02765527362 1.0134784519 0.998280021213 0.981755128787 0.967218261288 ... (400 elements, 20x20)]
  f_mdot_air_corr.DataType = 'double'
  f_mdot_air_corr.Complexity = 'real'
  f_mdot_air_corr.Dimensions = [20 20]
  f_mdot_air_corr_ld_bpt = Simulink.Parameter
  f_mdot_air_corr_ld_bpt.Value = [0.223381333333 0.285105122807 0.346828912281 0.408552701754 0.470276491228 0.532000280702 0.593724070175 0.655447859649 0.717171649123 0.778895438596 0.84061922807 0.902343017544 0.964066807018 1.02579059649 1.08751438596 1.14923817544 1.21096196491 1.27268575439 1.33440954386 1.39613333333]
  f_mdot_air_corr_ld_bpt.DataType = 'double'
  f_mdot_air_corr_ld_bpt.Complexity = 'real'
  f_mdot_air_corr_ld_bpt.Dimensions = [1 20]
  f_mdot_air_n_bpt = Simulink.Parameter
  f_mdot_air_n_bpt.Value = [750 973.6842 1197.3684 1421.0526 1644.7368 1868.4211 2092.1053 2315.7895 2539.4737 2763.1579 2986.8421 3210.5263 3434.2105 3657.8947 3881.5789 4105.2632 4328.9474 4552.6316 4776.3158 5000]
  f_mdot_air_n_bpt.DataType = 'double'
  f_mdot_air_n_bpt.Complexity = 'real'
  f_mdot_air_n_bpt.Dimensions = [1 20]
  f_mdot_intk = Simulink.Parameter
  f_mdot_intk.Value = [0 0 0 0 0 0 0 0 0 0 0 0 ... (400 elements, 20x20)]
  f_mdot_intk.DataType = 'double'
  f_mdot_intk.Complexity = 'real'
  f_mdot_intk.Dimensions = [20 20]
  f_mdot_intk_ecp_bpt = Simulink.Parameter
  f_mdot_intk_ecp_bpt.Value = [0 2.6316 5.2632 7.8947 10.5263 13.1579 15.7895 18.4211 21.0526 23.6842 26.3158 28.9474 31.5789 34.2105 36.8421 39.4737 42.1053 44.7368 47.3684 50]
  f_mdot_intk_ecp_bpt.DataType = 'double'
  f_mdot_intk_ecp_bpt.Complexity = 'real'
  f_mdot_intk_ecp_bpt.Dimensions = [1 20]
  f_mdot_trpd_bpt = Simulink.Parameter
  f_mdot_trpd_bpt.Value = [0 5.7895 11.5789 17.3684 23.1579 28.9474 34.7368 40.5263 46.3158 52.1053 57.8947 63.6842 69.4737 75.2632 81.0526 86.8421 92.6316 98.4211 104.2105 110]
  f_mdot_trpd_bpt.DataType = 'double'
  f_mdot_trpd_bpt.Complexity = 'real'
  f_mdot_trpd_bpt.Dimensions = [1 20]
  f_nv = Simulink.Parameter
  f_nv.Value = [0.64175366561 0.641419295169 0.640125365558 0.638690556197 0.644169906538 0.669178791311 0.731659452876 0.750078238889 0.750078238889 0.750078238889 0.750078238889 0.750078238889 ... (225 elements, 15x15)]
  f_nv.DataType = 'double'
  f_nv.Complexity = 'real'
  f_nv.Dimensions = [15 15]
  f_nv_n_bpt = Simulink.Parameter
  f_nv_n_bpt.Value = [750 1053.57142857 1357.14285714 1660.71428571 1964.28571429 2267.85714286 2571.42857143 2875 3178.57142857 3482.14285714 3785.71428571 4089.28571429 4392.85714286 4696.42857143 5000]
  f_nv_n_bpt.DataType = 'double'
  f_nv_n_bpt.Complexity = 'real'
  f_nv_n_bpt.Dimensions = [1 15]
  f_nv_prs_bpt = Simulink.Parameter
  f_nv_prs_bpt.Value = [31 40.6428571429 50.2857142857 59.9285714286 69.5714285714 79.2142857143 88.8571428571 98.5 108.142857143 117.785714286 127.428571429 137.071428571 146.714285714 156.357142857 166]
  f_nv_prs_bpt.DataType = 'double'
  f_nv_prs_bpt.Complexity = 'real'
  f_nv_prs_bpt.Dimensions = [1 15]
  f_sa = Simulink.Parameter
  f_sa.Value = [9.05 9.05 16.4373253582 15.3405265461 13.6074880273 9.83352189562 3.89388784387 0 0 0 0 0 ... (240 elements, 16x15)]
  f_sa.DataType = 'double'
  f_sa.Complexity = 'real'
  f_sa.Dimensions = [16 15]
  f_sa_ld_bpt = Simulink.Parameter
  f_sa_ld_bpt.Value = [0 0.2 0.275 0.35 0.425 0.5 0.575 0.65 0.725 0.8 0.875 0.95 1.025 1.1 1.175 1.25]
  f_sa_ld_bpt.DataType = 'double'
  f_sa_ld_bpt.Complexity = 'real'
  f_sa_ld_bpt.Dimensions = [1 16]
  f_sa_n_bpt = Simulink.Parameter
  f_sa_n_bpt.Value = [750 1053.57142857 1357.14285714 1660.71428571 1964.28571429 2267.85714286 2571.42857143 2875 3178.57142857 3482.14285714 3785.71428571 4089.28571429 4392.85714286 4696.42857143 5000]
  f_sa_n_bpt.DataType = 'double'
  f_sa_n_bpt.Complexity = 'real'
  f_sa_n_bpt.Dimensions = [1 15]
  f_sa_opt = Simulink.Parameter
  f_sa_opt.Value = [9.05 9.05 16.4373253582 15.3405265461 13.6074880273 9.83352189562 3.89388784387 2.22044604925e-16 2.22044604925e-16 2.22044604925e-16 2.22044604925e-16 2.22044604925e-16 ... (272 elements, 16x17)]
  f_sa_opt.DataType = 'double'
  f_sa_opt.Complexity = 'real'
  f_sa_opt.Dimensions = [16 17]
  f_startup_ect_bpt = Simulink.Parameter
  f_startup_ect_bpt.Value = [-40 0 20 50]
  f_startup_ect_bpt.DataType = 'double'
  f_startup_ect_bpt.Complexity = 'real'
  f_startup_ect_bpt.Dimensions = [1 4]
  f_startup_lambda_delta = Simulink.Parameter
  f_startup_lambda_delta.Value = [0.5 0.3 0.2 0]
  f_startup_lambda_delta.DataType = 'double'
  f_startup_lambda_delta.Complexity = 'real'
  f_startup_lambda_delta.Dimensions = [1 4]
  f_startup_lambda_delta_timecnst = Simulink.Parameter
  f_startup_lambda_delta_timecnst.Value = [90 40 12 0]
  f_startup_lambda_delta_timecnst.DataType = 'double'
  f_startup_lambda_delta_timecnst.Complexity = 'real'
  f_startup_lambda_delta_timecnst.Dimensions = [1 4]
  f_t_exh = Simulink.Parameter
  f_t_exh.Value = [739.936218766 750.584766028 772.770773797 791.235245621 803.106549716 885.862998064 920.498479307 920.498479307 920.498479307 920.498479307 920.498479307 920.498479307 ... (225 elements, 15x15)]
  f_t_exh.DataType = 'double'
  f_t_exh.Complexity = 'real'
  f_t_exh.Dimensions = [15 15]
  f_t_exh_l_bpt = Simulink.Parameter
  f_t_exh_l_bpt.Value = [0.2 0.275 0.35 0.425 0.5 0.575 0.65 0.725 0.8 0.875 0.95 1.025 1.1 1.175 1.25]
  f_t_exh_l_bpt.DataType = 'double'
  f_t_exh_l_bpt.Complexity = 'real'
  f_t_exh_l_bpt.Dimensions = [1 15]
  f_t_exh_n_bpt = Simulink.Parameter
  f_t_exh_n_bpt.Value = [750 1053.57142857 1357.14285714 1660.71428571 1964.28571429 2267.85714286 2571.42857143 2875 3178.57142857 3482.14285714 3785.71428571 4089.28571429 4392.85714286 4696.42857143 5000]
  f_t_exh_n_bpt.DataType = 'double'
  f_t_exh_n_bpt.Complexity = 'real'
  f_t_exh_n_bpt.Dimensions = [1 15]
  f_tap = Simulink.Parameter
  f_tap.Value = [0 0.526932471367 0.769562920372 0.98216383526 1.23343075188 1.55068263762 2.00046959085 2.58135491039 2.62499999998 2.62499999998 2.62499999998 2.62499999998 ... (315 elements, 21x15)]
  f_tap.DataType = 'double'
  f_tap.Complexity = 'real'
  f_tap.Dimensions = [21 15]
  f_tap_ld_bpt = Simulink.Parameter
  f_tap_ld_bpt.Value = [0 0.2 0.268421052632 0.336842105263 0.405263157895 0.473684210526 0.542105263158 0.610526315789 0.678947368421 0.747368421053 0.815789473684 0.884210526316 0.952631578947 1.02105263158 1.08947368421 1.15789473684 1.22631578947 1.29473684211 1.36315789474 1.43157894737 1.5]
  f_tap_ld_bpt.DataType = 'double'
  f_tap_ld_bpt.Complexity = 'real'
  f_tap_ld_bpt.Dimensions = [1 21]
  f_tap_n_bpt = Simulink.Parameter
  f_tap_n_bpt.Value = [750 1053.57142857 1357.14285714 1660.71428571 1964.28571429 2267.85714286 2571.42857143 2875 3178.57142857 3482.14285714 3785.71428571 4089.28571429 4392.85714286 4696.42857143 5000]
  f_tap_n_bpt.DataType = 'double'
  f_tap_n_bpt.Complexity = 'real'
  f_tap_n_bpt.Dimensions = [1 15]
  f_tm_corr = Simulink.Parameter
  f_tm_corr.Value = [0.839360054391 0.833393271885 0.82629554201 0.818442814437 0.811524387436 0.809164184856 0.814606352881 0.826887956871 0.842304598924 0.856886829014 0.869487025783 0.880530414174 ... (400 elements, 20x20)]
  f_tm_corr.DataType = 'double'
  f_tm_corr.Complexity = 'real'
  f_tm_corr.Dimensions = [20 20]
  f_tm_corr_n_bpt = Simulink.Parameter
  f_tm_corr_n_bpt.Value = [750 973.6842 1197.3684 1421.0526 1644.7368 1868.4211 2092.1053 2315.7895 2539.4737 2763.1579 2986.8421 3210.5263 3434.2105 3657.8947 3881.5789 4105.2632 4328.9474 4552.6316 4776.3158 5000]
  f_tm_corr_n_bpt.DataType = 'double'
  f_tm_corr_n_bpt.Complexity = 'real'
  f_tm_corr_n_bpt.Dimensions = [1 20]
  f_tm_corr_nd_bpt = Simulink.Parameter
  f_tm_corr_nd_bpt.Value = [0.3 0.38947 0.47895 0.56842 0.65789 0.74737 0.83684 0.92632 1.0158 1.1053 1.1947 1.2842 1.3737 1.4632 1.5526 1.6421 1.7316 1.8211 1.9105 2]
  f_tm_corr_nd_bpt.DataType = 'double'
  f_tm_corr_nd_bpt.Complexity = 'real'
  f_tm_corr_nd_bpt.Dimensions = [1 20]
  f_tpp = Simulink.Parameter
  f_tpp.Value = [0 100]
  f_tpp.DataType = 'double'
  f_tpp.Complexity = 'real'
  f_tpp.Dimensions = [1 2]
  f_tpp_tap_bpt = Simulink.Parameter
  f_tpp_tap_bpt.Value = [0 100]
  f_tpp_tap_bpt.DataType = 'double'
  f_tpp_tap_bpt.Complexity = 'real'
  f_tpp_tap_bpt.Dimensions = [1 2]
  f_tq_fric = Simulink.Parameter
  f_tq_fric.Value = [-100  0  4.16  4.8  5.44  6.05  6.64  7.23  7.81  8.39  8.97  9.54  10.1  10.7  11.3  11.9  12.5; -100  0  4.16  4.8  5.44  6.05  6.64  7.23  7.81  8.39  8.97  9.54  10.1  10.7  11.3  11.9  12.5; -100  0  4.42  5.07  5.69  6.29  6.89  7.49  8.09  8.69  9.28  9.86  10.4  11  11.6  12.2  12.8; -100  0  4.69  5.36  5.98  6.58  7.18  7.79  8.41  9.02  9.62  10.2  10.8  11.4  11.9  12.5  13.1; -100  0  4.88  5.59  6.25  6.87  7.48  8.09  8.71  9.32  9.92  10.5  11.1  11.7  12.3  12.9  13.4; -100  0  4.94  5.74  6.45  7.12  7.75  8.37  8.99  9.59  10.2  10.8  11.4  11.9  12.6  13.2  13.8; -100  0  4.93  5.76  6.56  7.29  7.97  8.62  9.23  9.83  10.4  11  11.6  12.2  12.8  13.4  14.1; -100  0  4.85  5.67  6.57  7.37  8.11  8.8  9.43  10  10.6  11.2  11.8  12.4  13  13.7  14.3; -100  0  4.74  5.57  6.46  7.34  8.14  8.88  9.55  10.2  10.8  11.4  12  12.6  13.2  13.8  14.4; -100  0  4.63  5.42  6.27  7.19  8.05  8.83  9.55  10.2  10.9  11.5  12.1  12.7  13.3  14  14.6; -100  0  4.52  5.29  6.11  6.98  7.84  8.65  9.4  10.1  10.8  11.5  12.1  12.8  13.4  14.1  14.6; -100  0  4.42  5.18  5.97  6.79  7.6  8.39  9.15  9.88  10.6  11.3  12.1  12.8  13.5  14.1  14.7; -100  0  4.34  5.09  5.86  6.64  7.42  8.17  8.88  9.6  10.3  11.1  11.9  12.7  13.4  14.1  14.7; -100  0  4.27  5.01  5.76  6.52  7.28  8.03  8.74  9.39  10.1  10.8  11.6  12.4  13.2  14  14.7; -100  0  4.21  4.94  5.67  6.42  7.16  7.89  8.59  9.25  9.93  10.7  11.5  12.3  13.1  13.8  14.6; -100  0  4.15  4.87  5.6  6.33  7.06  7.77  8.47  9.14  9.84  10.6  11.3  12.1  12.9  13.7  14.4]
  f_tq_fric.DataType = 'double'
  f_tq_fric.Complexity = 'real'
  f_tq_fric.Dimensions = [16 17]
  f_tq_inr : Simulink.Parameter (value not decoded)
  f_tq_inr_l_bpt : Simulink.Parameter (value not decoded)
  f_tq_inr_n_bpt : Simulink.Parameter (value not decoded)
  f_tq_nl : Simulink.Parameter (value not decoded)
  f_tq_nl_l_bpt : Simulink.Parameter (value not decoded)
  f_tq_nl_n_bpt : Simulink.Parameter (value not decoded)
  f_tq_pump : Simulink.Parameter (value not decoded)
  f_vivc : Simulink.Parameter (value not decoded)
  f_vivc_icp_bpt : Simulink.Parameter (value not decoded)
  f_wap : Simulink.Parameter (value not decoded)
  f_wap_ld_bpt : Simulink.Parameter (value not decoded)
  f_wap_n_bpt : Simulink.Parameter (value not decoded)
  g = Simulink.Parameter
  g.Value = 9.81
  g.DataType = 'double'
  g.Complexity = 'real'
  g.Dimensions = [1 1]
  grEff : Simulink.Parameter (value not decoded)
  h : Simulink.Parameter (value not decoded)
  k : Simulink.Parameter (value not decoded)
  k1 : Simulink.Parameter (value not decoded)
  k2 : Simulink.Parameter (value not decoded)
  kappamax : Simulink.Parameter (value not decoded)
  lam_x : Simulink.Parameter (value not decoded)
  mu_kinetic : Simulink.Parameter (value not decoded)
  mu_static : Simulink.Parameter (value not decoded)
  muc : Simulink.Parameter (value not decoded)
  muk : Simulink.Parameter (value not decoded)
  mus : Simulink.Parameter (value not decoded)
  num_pads : Simulink.Parameter (value not decoded)
  omega1_c : Simulink.Parameter (value not decoded)
  omega2_c : Simulink.Parameter (value not decoded)
  omega_bpts : Simulink.Parameter (value not decoded)
  omega_c : Simulink.Parameter (value not decoded)
  omega_o : Simulink.Parameter (value not decoded)
  omega_o_J : Simulink.Parameter (value not decoded)
  omegai_o : Simulink.Parameter (value not decoded)
  omegain_o : Simulink.Parameter (value not decoded)
  omegal : Simulink.Parameter (value not decoded)
  omegao : Simulink.Parameter (value not decoded)
  omegaout_o : Simulink.Parameter (value not decoded)
  omegat_o : Simulink.Parameter (value not decoded)
  omegau : Simulink.Parameter (value not decoded)
  omegaw1o : Simulink.Parameter (value not decoded)
  omegaw2o : Simulink.Parameter (value not decoded)
  phi : Simulink.Parameter (value not decoded)
  philu : Simulink.Parameter (value not decoded)
  power_max : Simulink.Parameter (value not decoded)
  press : Simulink.Parameter (value not decoded)
  psi : Simulink.Parameter (value not decoded)
  q_o : Simulink.Parameter (value not decoded)
  tauC : Simulink.Parameter (value not decoded)
  tauC_1 : Simulink.Parameter (value not decoded)
  tauC_LSD : Simulink.Parameter (value not decoded)
  tauTC : Simulink.Parameter (value not decoded)
  tau_egr : Simulink.Parameter (value not decoded)
  tau_s : Simulink.Parameter (value not decoded)
  tc : Simulink.Parameter (value not decoded)
  theta_o : Simulink.Parameter (value not decoded)
  theta_o_Veh : Simulink.Parameter (value not decoded)
  torque_max : Simulink.Parameter (value not decoded)
  ts : Simulink.Parameter (value not decoded)
  w1_o : Simulink.Parameter (value not decoded)
  w_eff_bp : Simulink.Parameter (value not decoded)
  wc : Simulink.Parameter (value not decoded)
  win_o : Simulink.Parameter (value not decoded)
  wout_o : Simulink.Parameter (value not decoded)
  x_o : Simulink.Parameter (value not decoded)
  xdot_o : Simulink.Parameter (value not decoded)
  z_o : Simulink.Parameter (value not decoded)
  zdot_o : Simulink.Parameter (value not decoded)
  zeta : Simulink.Parameter (value not decoded)
symbols that are objects in the model workspace (value not decoded): k, w_eff_bp
undefined symbols (not defined in the file or in its folder): Lock, up
libraries: autolibpowerinfoutils x5, autolibsharedcoupling x4, autolibshared x3, autolibutils x2, autolibshareddiff x2, autolibsharedmappedengines x1, autolibdcdc x1, autolibdatasheetbattery x1, autolibmappedmotor x1, autolibsharedtransfixedgear x1, autolibtrqconv x1
(part 1 of 3)
settings Model: Creator=omert  LastModifiedBy=omert

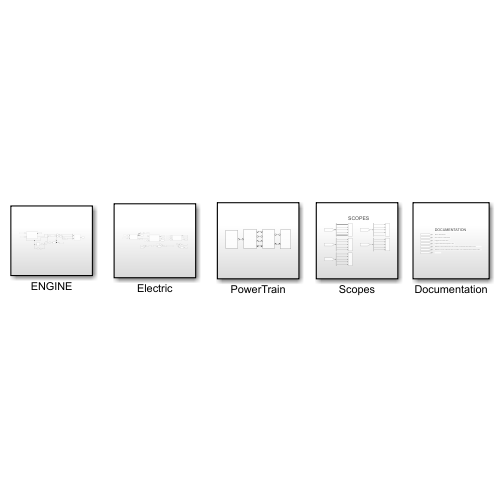
[thumbnail: Simulink's stored preview of the top-level diagram]
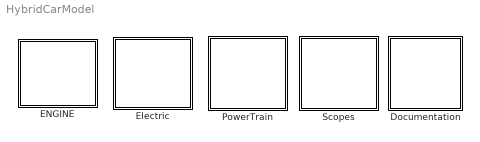
== system HybridCarModel ==
  Documentation : Subsystem
  ENGINE : Subsystem
  Electric : Subsystem
  PowerTrain : Subsystem
  Scopes : Subsystem

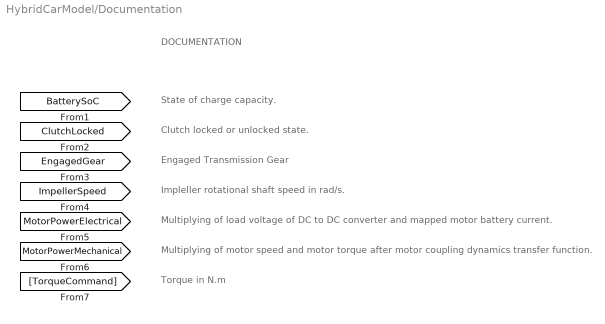
== system HybridCarModel/Documentation ==
  note: Clutch locked or unlocked state.
  note: Torque in N.m
  note: DOCUMENTATION
  note: State of charge capacity.
  note: Engaged Transmission Gear
  note: Impleller rotational shaft speed in rad/s.
  note: Multiplying of motor speed and motor torque after motor coupling dynamics transfer function.
  note: Multiplying of load voltage of DC to DC converter and mapped motor battery current.

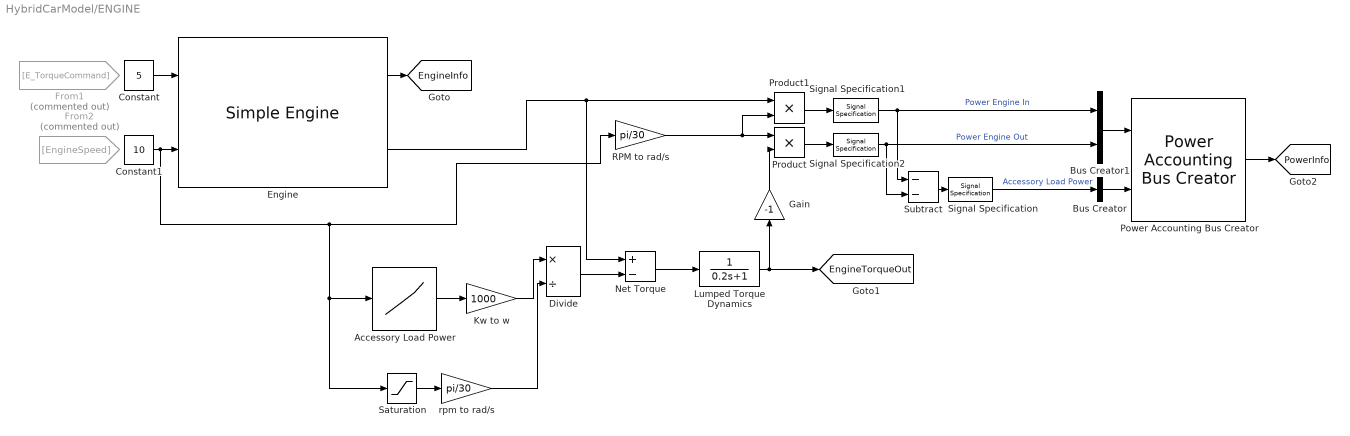
== system HybridCarModel/ENGINE ==
  Accessory Load Power : Lookup_n-D  NumberOfTableDimensions=1  LookupTableObject=''  BreakpointsForDimension1=[300 750]  Table=[0 0]  ExtrapMethod=Clip  InternalRulePriority=Speed  RndMeth=Simplest
  Bus Creator : BusCreator  Inputs=1
  Bus Creator1 : BusCreator  Inputs=2
  Constant : Constant  Value=5
  Constant1 : Constant  Value=10
  Divide : Product  Inputs=*/
  Engine : autolibsharedmappedengines/Simple Engine  f_tqmax=[75.679776480773256 75.679776480773256 97.173658538143172 116.84042599160529 152.21029882684542 175 174.99889520597083 174.99996520122858 175 175 175 175 175 175 175 175]  f_tqmax_n_bpt=[0 750 1053.57142857143 1357.14285714286 1660.71428571429 1964.28571428571 2267.85714285714 2571.42857142857 2875 3178.57142857143 3482.14285714286 3785.71428571429 4089.28571428571 4392.85714285714 4696.42857142857 5000]  Lhv=46e6  Sg=0.745  BsfcAvg=350  aMode=1
      settings: LibrarySourceBlock=autolibenginesystems/Simple Engine
  From1 : From  Commented=on  GotoTag=E_TorqueCommand
  From2 : From  Commented=on  GotoTag=EngineSpeed
  Gain : Gain  Gain=-1
  Kw to w : Gain  Gain=1000
  Lumped Torque Dynamics : TransferFcn  Denominator=[0.2 1]
  Net Torque : Sum  Inputs=+-
  Power Accounting Bus Creator : autolibpowerinfoutils/Power Accounting Bus Creator  AssctBlkSelPopup=Parent  RefBlkName='libraryname/blkname'  PwrTrnsfrdCheckBox=on  PwrNotTrnsfrdCheckBox=on  PwrStoredCheckBox=off  aMode=aMode
  Product : Product
  Product1 : Product
  RPM to rad/s : Gain  Gain=pi/30
  Saturation : Saturate  UpperLimit=Inf  LowerLimit=300  ZeroCross=off
  Signal Specification : SignalSpecification  Unit=W
  Signal Specification1 : SignalSpecification  Unit=W
  Signal Specification2 : SignalSpecification  Unit=W
  Subtract : Sum  Inputs=--
  rpm to rad/s : Gain  Gain=pi/30
  tag scope: EngineInfo=global, EngineTorqueOut=global, PowerInfo=global
  wires:
  Accessory Load Power/1 -> Kw to w/1
  Subtract/1 -> Signal Specification/1
  Constant1/1 -> RPM to rad/s/1, Saturation/1, Accessory Load Power/1, Engine/2
  rpm to rad/s/1 -> Divide/2
  Signal Specification2/1 -> Subtract/2, Bus Creator1/2  "Power Engine Out"
  Bus Creator/1 -> Power Accounting Bus Creator/2
  Engine/1 -> [EngineInfo]
  Kw to w/1 -> Divide/1
  Product1/1 -> Signal Specification1/1
  Engine/2 -> Product1/1, Net Torque/1
  Product/1 -> Signal Specification2/1
  Saturation/1 -> rpm to rad/s/1
  Signal Specification/1 -> Bus Creator/1  "Accessory Load Power"
  Divide/1 -> Net Torque/2
  Lumped Torque Dynamics/1 -> [EngineTorqueOut], Gain/1
  Power Accounting Bus Creator/1 -> [PowerInfo]
  Net Torque/1 -> Lumped Torque Dynamics/1
  Bus Creator1/1 -> Power Accounting Bus Creator/1
  Gain/1 -> Product/2
  RPM to rad/s/1 -> Product1/2, Product/1
  Signal Specification1/1 -> Subtract/1, Bus Creator1/1  "Power Engine In"
  Constant/1 -> Engine/1

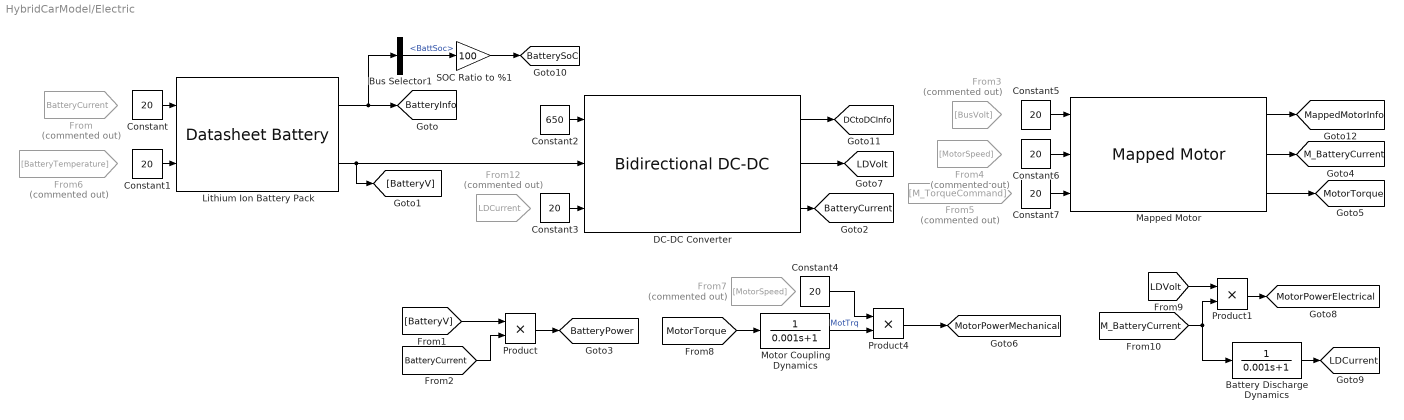
== system HybridCarModel/Electric ==
  Battery Discharge Dynamics : TransferFcn  Denominator=[0.001 1]
  Bus Selector1 : BusSelector  OutputSignals=BattSoc
  Constant{,1,3..7} (7 alike) : Constant  Value=20
  Constant2 : Constant  Value=650
  DC-DC Converter : autolibdcdc/Bidirectional DC-DC  Tc=Tc  Vinit=Vinit  Plimit=Plimit  param_loss=Single efficiency measurement  eff=eff  v_loss_bp=[0 200 400 600 800 1000]  i_loss_bp=[0 25 50 75 100]  losses_table=[100 100 100 100 100;100 150 200 250 300;100 200 300 400 500;100 250 400 550 700;100 300 500 700 900;100 350 600 850 1100]  v_eff_bp=[200 400 600 800 1000]  i_eff_bp=[25 50 75 100]  efficiency_table=[96.2 98.1 98.7 99;98.1 99 99.4 99.5;98.7 99.4 99.6 99.7;99 99.5 99.7 99.8;99.2 99.6 99.7 99.8]  x_v_bp=[-1000 -800 -600 -400 -200 200 400 600 800 1000]  x_i_bp=[-100 -75 -50 -25 25 50 75 100]  x_losses_mat=[200.400801603196 225.67703109328 200.803212851408 201.612903225806 199.999999999997 200 225 200;160.320641282556 180.541624874624 201.005025125625 202.020202020203 200 200 180 160;180.541624874624 180.722891566267 181.086519114686 197.568389057748 194.999999999999 179.999999999997 180 180;201.005025125625 181.086519114686 202.020202020203 193.67991845056 190 200 179.999999999997 200;202.020202020203 197.568389057748 193.67991845056 197.505197505197 190 190 194.999999999999 200;200 194.999999999999 190 190 197.505197505197 193.67991845056 197.568389057748 202.020202020203;200 179.999999999997 200 190 193.67991845056 202.020202020203 181.086519114686 201.005025125625;180 180 179.999999999997 194.999999999999 197.568389057748 181.086519114686 180.722891566267 180.541624874624;160 180 200 200 202.020202020203 201.005025125625 180.541624874624 160.320641282556;200 225 200 199.999999999997 201.612903225806 200.803212851408 225.67703109328 200.400801603196]  RefBlkName='autolibdcdc/Bidirectional DC-DC'  CalLossMapData={'BaseCageProjectFileName','';'BaseMbcProjectFileName','';'TaskName','Calibrate Inverter Loss Map';'ChildTasks',{{'DataName','';'TaskName','Import Loss Data'},{'TaskName','Generate Response Models'},{'TaskName','Generate Calibration'},{'TaskName','Update Block Parameters'}}}
  From : From  Commented=on  GotoTag=BatteryCurrent  TagVisibility=global
  From12 : From  Commented=on  GotoTag=LDCurrent  TagVisibility=global
  From3 : From  Commented=on  GotoTag=BusVolt
  From4 : From  Commented=on  GotoTag=MotorSpeed
  From5 : From  Commented=on  GotoTag=M_TorqueCommand
  From6 : From  Commented=on  GotoTag=BatteryTemperature
  From7 : From  Commented=on  GotoTag=MotorSpeed
  Lithium Ion Battery Pack : autolibdatasheetbattery/Datasheet Battery  CapacityCtrl=Parameter  OutputVlt=Filtered  BattChargeMax=5.3  Em=Em  CapLUTBp=CapLUTBp  RInt=RInt  BattTempBp=BattTempBp  CapSOCBp=CapSOCBp  Ns=72  Np=1  BattCapInit=3.18  Tc=0.001  Vinit=Ns*interp1(CapLUTBp, Em, BattCapInit/BattChargeMax)  RefBlkName='autolibdatasheetbattery/Datasheet Battery'
  Mapped Motor : autolibmappedmotor/Mapped Motor  port_config=Speed  param_by=Tabulated torque-speed envelope  w_t=w_eff_bp.*pi/30  T_t=T_t  torque_max=torque_max  power_max=power_max  Tc=0.02  param_loss=Tabulated efficiency data  eff=100  w_eff=375  T_eff=0.08  Piron=0  Pbase=0  w_eff_bp=w_eff_bp.*pi/30  T_eff_bp=T_eff_bp  Temp_eff_bp=[233.15 293.15 373.15]  losses_table=[1 2;3 4]  losses_table_3d=cat(3,1.05*[1.49 1.67 2.21 3.10; 0.42 0.69 1.14 2.03; 0.06 0.24 0.78 1.68; 0.42 0.69 1.14 2.03; 1.49 1.67 2.21 3.10],[1.49 1.67 2.21 3.10; 0.42 0.69 1.14 2.03; 0.06 0.24 0.78 1.68; 0.42 0.69 1.14 2.03; 1.49 1.67 2.21 3.10],1.03*[1.49 1.67 2.21 3.10; 0.42 0.69 1.14 2.03; 0.06 0.24 0.78 1.68; 0.42 0.69 1.14 2.03; 1.49 1.67 2.21 3.10])  efficiency_table=efficiency_table  efficiency_table_3d=cat(3,90*ones(5,4),95*ones(5,4),92*ones(5,4))  J=5e-6  b=1e-5  omega_o=0  T_t_extended=[47.74648293 52.08707228 57.29577951 63.66197724 71.61972439 81.85111359 95.49296586 114.591559 143.2394488 190.9859317 200 200 200 200 200 200 200 190.9859317 143.2394488 114.591559 95.49296586 81.85111359 71.61972439 63.66197724 57.29577951 52.08707228 47.74648293]  w_t_extended=[-628.318530717959 -575.958653158129 -523.598775598299 -471.238898038469 -418.879020478639 -366.519142918809 -314.159265358979 -261.799387799149 -209.43951023932 -157.07963267949 -149.999649206931 -104.71975511966 -52.3598775598299 0 52.3598775598299 104.71975511966 149.999649206931 157.07963267949 209.43951023932 261.799387799149 314.159265358979 366.519142918809 418.879020478639 471.238898038469 523.598775598299 575.958653158129 628.318530717959]  KLossIron=0  KLossCopper=0  x_w_eff_vec=[-628.318530717959 -575.958653158129 -523.598775598299 -471.238898038469 -418.879020478639 -366.519142918809 -314.159265358979 -261.799387799149 -209.43951023932 -157.07963267949 -149.999649206931 -104.71975511966 -52.3598775598299 0 52.3598775598299 104.71975511966 149.999649206931 157.07963267949 209.43951023932 261.799387799149 314.159265358979 366.519142918809 418.879020478639 471.238898038469 523.598775598299 575.958653158129 628.318530717959]  x_T_eff_vec=[-200 -180 -160 -140 -120 -100 -80 -60 -40 -20 0 20 40 60 80 100 120 140 160 180 200]  x_tmp_eff_vec=[233.15 293.15 373.15]  x_losses_mat=[9458.558526937 8512.7026742433 7566.8468215496 6620.9909688559 5675.1351161622 4729.2792634685 3783.4234107748 2837.5675580811 2485.6557259172 2045.68823954684 0 1759.29188601028 2261.94671058465 2638.93782901542 3518.58377202057 4398.22971502571 5277.87565803085 6157.52160103599 7037.16754404113 7916.81348704627 8796.45943005141;8670.34531635892 7803.31078472303 6936.27625308713 6069.24172145124 5202.20718981535 4335.17265817946 3468.13812654357 2601.10359490768 2003.3344457674 1875.21421958461 0 1612.68422884276 1843.06769010601 2419.02634326414 3225.36845768552 4031.7105721069 4838.05268652828 5644.39480094966 6450.73691537104 7257.07902979242 8063.4211442138;7882.13210578084 7093.91889520275 6305.70568462467 5517.49247404659 4729.2792634685 3941.06605289042 3152.85284231233 2364.63963173425 1821.21313251582 1704.74019962237 0 1466.07657167524 1675.51608191456 2199.11485751285 2932.15314335047 3665.19142918809 4398.22971502571 5131.26800086333 5864.30628670094 6597.34457253856 7330.38285837618;7093.91889520275 6384.52700568248 5675.1351161622 4965.74322664193 4256.35133712165 3546.95944760138 2837.5675580811 2128.17566856083 1864.2417944379 1534.26617966013 0 1319.46891450771 1696.46003293849 1979.20337176157 2638.93782901542 3298.67228626928 3958.40674352314 4618.14120077699 5277.87565803085 5937.61011528471 6597.34457253856;6305.70568462467 5675.1351161622 5044.56454769974 4413.99397923727 3783.4234107748 3152.85284231233 2522.28227384987 1891.7117053874 1657.10381727813 1363.7921596979 0 1172.86125734019 1507.9644737231 1759.29188601028 2345.72251468038 2932.15314335047 3518.58377202057 4105.01440069066 4691.44502936075 5277.87565803085 5864.30628670094;5517.49247404658 4965.74322664193 4413.99397923727 3862.24473183261 3310.49548442795 2758.74623702329 2549.69838552215 1912.27378914161 1628.97396852804 1396.26340159546 0 1172.86125734019 1466.07657167524 1759.29188601028 2345.72251468038 2565.63400043166 3078.76080051799 3591.88760060433 4105.01440069066 4618.14120077699 5131.26800086332;4729.2792634685 4256.35133712165 3783.4234107748 3310.49548442795 2837.5675580811 2731.81969877373 2485.6557259172 1864.2417944379 1713.59599286716 1379.23579913698 0 1130.97335529233 1507.9644737231 1696.46003293849 2261.94671058465 2513.27412287183 2638.93782901542 3078.760800518 3518.58377202057 3958.40674352314 4398.22971502571;5178.44942899416 4660.60448609474 3642.42626503164 3187.12298190269 2731.81969877373 2589.22471449708 2071.37977159766 1745.32925199433 1427.99666072263 1149.36316594749 0 942.477796076938 1256.63706143592 1570.7963267949 1884.95559215388 2356.19449019234 2513.27412287183 2932.15314335047 3351.03216382911 4241.15008234622 4712.38898038469;5711.98664289054 5140.78797860148 4569.58931431243 3257.94793705608 2792.52680319093 2327.10566932577 1861.68453546062 1713.59599286716 1363.7921596979 1047.1975511966 0 837.758040957278 1172.86125734019 1507.9644737231 1675.51608191456 2094.39510239319 2513.27412287183 2932.15314335047 4021.23859659494 4523.8934211693 5026.54824574367;5114.22059886711 4602.7985389804 4091.37647909369 2998.79298751753 2570.39398930074 2141.99499108395 1713.59599286716 1285.19699465037 1022.84411977342 785.398163397448 0 628.318530717959 879.645943005142 1130.97335529233 1507.9644737231 1884.95559215388 2261.94671058465 2638.93782901543 3518.58377202057 3958.40674352314 4398.22971502571;5714.27235074022 5142.8451156662 3906.96760725029 3418.596656344 2454.53971429523 2045.44976191269 1636.35980953016 1465.11285271886 976.741901812573 749.998246034654 0 599.998596827723 839.998035558812 1259.99705333822 1439.99663238654 1799.99579048317 2159.9949485798 2939.99312445584 3359.99214223525 4319.98989715961 4799.98877462179;4597.45266378994 4137.70739741095 3191.45920364677 2792.52680319093 2045.68823954684 1704.74019962237 1363.7921596979 1022.84411977342 797.864800911693 590.726823751927 0 460.766922526503 670.206432765823 879.645943005142 1172.86125734019 1466.07657167524 1759.29188601028 ...(+4852 chars)]  x_losses_mat_3d=cat(3,[3.255 2.3205 1.7535 1.5645 1.7535 2.3205 3.255;2.1315 1.197 0.7245 0.441 0.7245 1.197 2.1315;1.764 0.819 0.252 0.063 0.252 0.819 1.764;2.1315 1.197 0.7245 0.441 0.7245 1.197 2.1315;3.255 2.3205 1.7535 1.5645 1.7535 2.3205 3.255],[3.1 2.21 1.67 1.49 1.67 2.21 3.1;2.03 1.14 0.69 0.42 0.69 1.14 2.03;1.68 0.78 0.24 0.06 0.24 0.78 1.68;2.03 1.14 0.69 0.42 0.69 1.14 2.03;3.1 2.21 1.67 1.49 1.67 2.21 3.1],[3.193 2.2763 1.7201 1.5347 1.7201 2.2763 3.193;2.0909 1.1742 0.7107 0.4326 0.7107 1.1742 2.0909;1.7304 0.8034 0.2472 0.0618 0.2472 0.8034 1.7304;2.0909 1.1742 0.7107 0.4326 0.7107 1.1742 2.0909;3.193 2.2763 1.7201 1.5347 1.7201 2.2763 3.193])  CalLossMapData={}  CalLossWithTempMapData={}  aMode=aMode  RefBlkName='autolibmappedmotor/Mapped Motor'
  Motor Coupling Dynamics : TransferFcn  Denominator=[0.001 1]
  Product : Product
  Product1 : Product
  Product4 : Product
  SOC Ratio to %1 : Gain  Gain=100
  tag scope: BatteryCurrent=global, BatteryInfo=global, BatteryPower=global, BatterySoC=global, DCtoDCInfo=global, LDCurrent=global, LDVolt=global, M_BatteryCurrent=global, MappedMotorInfo=global, MotorPowerElectrical=global, MotorPowerMechanical=global, MotorTorque=global
  wires:
  DC-DC Converter/3 -> [BatteryCurrent]
  Bus Selector1/1 -> SOC Ratio to %1/1  "<BattSoc>"
  DC-DC Converter/2 -> [LDVolt]
  Mapped Motor/3 -> [MotorTorque]
  SOC Ratio to %1/1 -> [BatterySoC]
  Constant2/1 -> DC-DC Converter/1
  Lithium Ion Battery Pack/2 -> DC-DC Converter/2, [BatteryV]
  DC-DC Converter/1 -> [DCtoDCInfo]
  Lithium Ion Battery Pack/1 -> [BatteryInfo], Bus Selector1/1
  Mapped Motor/2 -> [M_BatteryCurrent]
  Mapped Motor/1 -> [MappedMotorInfo]
  [BatteryV] -> Product/1
  [BatteryCurrent] -> Product/2
  Product/1 -> [BatteryPower]
  [MotorTorque] -> Motor Coupling Dynamics/1
  Motor Coupling Dynamics/1 -> Product4/2  "MotTrq"
  Product4/1 -> [MotorPowerMechanical]
  Product1/1 -> [MotorPowerElectrical]
  [LDVolt] -> Product1/1
  [M_BatteryCurrent] -> Battery Discharge Dynamics/1, Product1/2
  Battery Discharge Dynamics/1 -> [LDCurrent]
  Constant1/1 -> Lithium Ion Battery Pack/2
  Constant/1 -> Lithium Ion Battery Pack/1
  Constant3/1 -> DC-DC Converter/3
  Constant4/1 -> Product4/1
  Constant5/1 -> Mapped Motor/1
  Constant7/1 -> Mapped Motor/3
  Constant6/1 -> Mapped Motor/2

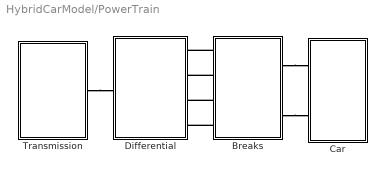
== system HybridCarModel/PowerTrain ==
  Breaks : Subsystem
  Car : Subsystem
  Differential : Subsystem
  Transmission : Subsystem
  connections:
  Transmission/RConn1 -- Differential/LConn1
  Breaks/LConn1 -- Differential/RConn1
  Breaks/LConn2 -- Differential/RConn2
  Breaks/LConn3 -- Differential/RConn3
  Breaks/LConn4 -- Differential/RConn4
  Breaks/RConn1 -- Car/LConn1
  Breaks/RConn2 -- Car/LConn2

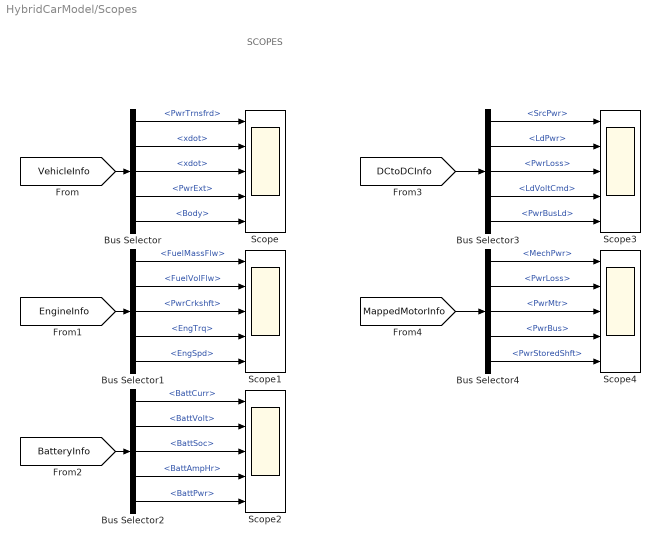
== system HybridCarModel/Scopes ==
  note: SCOPES
  Bus Selector : BusSelector  OutputSignals=PwrInfo.PwrTrnsfrd,BdyFrm.RearAxl.Vel.xdot,BdyFrm.FrntAxl.Vel.xdot,BdyFrm.Pwr.PwrExt,BdyFrm.Forces.Body
  Bus Selector1 : BusSelector  OutputSignals=FuelMassFlw,FuelVolFlw,PwrInfo.PwrTrnsfrd.PwrCrkshft,EngTrq,EngSpd
  Bus Selector2 : BusSelector  OutputSignals=BattCurr,BattVolt,BattSoc,BattAmpHr,BattPwr
  Bus Selector3 : BusSelector  OutputSignals=SrcPwr,LdPwr,PwrLoss,LdVoltCmd,PwrInfo.PwrTrnsfrd.PwrBusLd
  Bus Selector4 : BusSelector  OutputSignals=MechPwr,PwrLoss,PwrInfo.PwrTrnsfrd.PwrMtr,PwrInfo.PwrTrnsfrd.PwrBus,PwrInfo.PwrStored.PwrStoredShft
  Scope{,1..4} (5 alike) : Scope  NumInputPorts=5
  wires:
  Bus Selector/5 -> Scope/5  "<Body>"
  Bus Selector/1 -> Scope/1  "<PwrTrnsfrd>"
  [VehicleInfo] -> Bus Selector/1
  Bus Selector/2 -> Scope/2  "<xdot>"
  Bus Selector/3 -> Scope/3  "<xdot>"
  Bus Selector/4 -> Scope/4  "<PwrExt>"
  [EngineInfo] -> Bus Selector1/1
  Bus Selector1/1 -> Scope1/1  "<FuelMassFlw>"
  Bus Selector1/2 -> Scope1/2  "<FuelVolFlw>"
  Bus Selector1/3 -> Scope1/3  "<PwrCrkshft>"
  Bus Selector1/4 -> Scope1/4  "<EngTrq>"
  Bus Selector1/5 -> Scope1/5  "<EngSpd>"
  [BatteryInfo] -> Bus Selector2/1
  Bus Selector2/1 -> Scope2/1  "<BattCurr>"
  Bus Selector2/2 -> Scope2/2  "<BattVolt>"
  Bus Selector2/3 -> Scope2/3  "<BattSoc>"
  Bus Selector2/4 -> Scope2/4  "<BattAmpHr>"
  Bus Selector2/5 -> Scope2/5  "<BattPwr>"
  [DCtoDCInfo] -> Bus Selector3/1
  Bus Selector3/1 -> Scope3/1  "<SrcPwr>"
  Bus Selector3/2 -> Scope3/2  "<LdPwr>"
  Bus Selector3/3 -> Scope3/3  "<PwrLoss>"
  Bus Selector3/4 -> Scope3/4  "<LdVoltCmd>"
  Bus Selector3/5 -> Scope3/5  "<PwrBusLd>"
  [MappedMotorInfo] -> Bus Selector4/1
  Bus Selector4/1 -> Scope4/1  "<MechPwr>"
  Bus Selector4/2 -> Scope4/2  "<PwrLoss>"
  Bus Selector4/3 -> Scope4/3  "<PwrMtr>"
  Bus Selector4/4 -> Scope4/4  "<PwrBus>"
  Bus Selector4/5 -> Scope4/5  "<PwrStoredShft>"
